simulink model "first order system"  (R2021a)
settings: Solver=VariableStepAuto  StartTime=0.0  StopTime=42  RelTol=1e-3
settings Model: Creator=hritw  LastModifiedBy=hritw

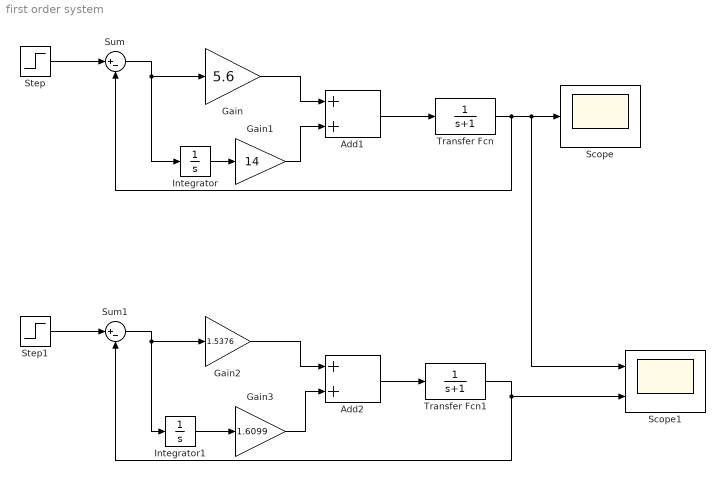
== system first order system ==
  Add1 : Sum
  Add2 : Sum
  Gain : Gain  Gain=5.6
  Gain1 : Gain  Gain=14
  Gain2 : Gain  Gain=1.5376
  Gain3 : Gain  Gain=1.6099
  Integrator : Integrator
  Integrator1 : Integrator
  Scope : Scope
  Scope1 : Scope  NumInputPorts=2
  Step : Step  SampleTime=0
  Step1 : Step  SampleTime=0
  Sum : Sum  Inputs=|+-
  Sum1 : Sum  Inputs=|+-
  Transfer Fcn : TransferFcn  Denominator=[1 1]
  Transfer Fcn1 : TransferFcn  Denominator=[1 1]
  wires:
  Add1/1 -> Transfer Fcn/1
  Gain/1 -> Add1/1
  Integrator/1 -> Gain1/1
  Gain1/1 -> Add1/2
  Transfer Fcn/1 -> Scope1/1, Scope/1, Sum/2
  Sum/1 -> Gain/1, Integrator/1
  Step/1 -> Sum/1
  Gain2/1 -> Add2/1
  Add2/1 -> Transfer Fcn1/1
  Gain3/1 -> Add2/2
  Integrator1/1 -> Gain3/1
  Step1/1 -> Sum1/1
  Sum1/1 -> Gain2/1, Integrator1/1
  Transfer Fcn1/1 -> Scope1/2, Sum1/2
